simulink model "openManipulatorTorqueCtrlTask"  (R2021a)
settings: Solver=VariableStepAuto  StartTime=0.0  StopTime=3  RelTol=1e-3
PreLoadFcn:
  | openManipulatorParameters;
undefined symbols (not defined in the file): ctrlLowerLimit, ctrlUpperLimit, gripLowerLimit, gripUpperLimit, initPos, Kd, KdCart, Kfilt, KfiltCart, KiCart, KiGrip, KpCart, KpGrip, robot, TsCtrl, X, Y, Z
libraries: nesl_utility x26, sm_lib x23, OpenManipulatorLib x7, fl_lib x4, pid_lib x3, robotmaniplib x2, Multibody_Multiphysics_Lib x2
(part 2 of 2)

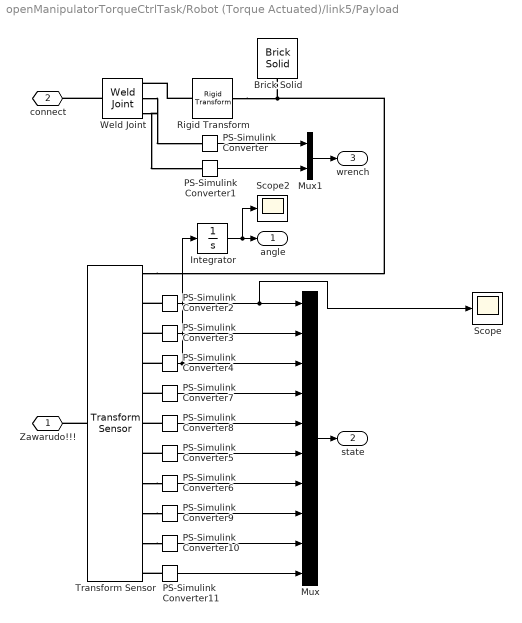
== system openManipulatorTorqueCtrlTask/Robot (Torque Actuated)/link5/Payload ==
  Brick Solid : sm_lib/Body Elements/Brick Solid  GraphicAmbientColor=[0.15 0.15 0.15 1.0]  BasedOnType=Density  BrickDimensions=[0.03 0.3 0.03]  BrickDimensionUnits=m  CenterOfMass=[0 0 0]  CenterOfMassUnits=m  GraphicDiffuseColor=[0.5 0.5 0.5]  Density=100  DensityUnits=kg/m^3  DoExposeReferenceFrame=on  GraphicEmissiveColor=[0.0 0.0 0.0 1.0]  ExportEntireGeometry=off  SerializedFrames=<Frames/>  MarkerShape=Sphere  MarkerSize=10  GraphicType=FromGeometry  InertiaType=CalculateFromGeometry  Mass=1  MassUnits=kg  MomentsOfInertia=[1 1 1]  MomentsOfInertiaUnits=kg*m^2  GraphicOpacity=1.0  ProductsOfInertia=[0 0 0]  ProductsOfInertiaUnits=kg*m^2  GraphicShininess=75  GraphicSpecularColor=[0.5 0.5 0.5 1.0]  GraphicVisPropType=SimpleVisualProperties
  Integrator : Integrator
  Mux : Mux  Inputs=10
  Mux1 : Mux  Inputs=2
  PS-Simulink Converter{,1..11} (12 alike) : nesl_utility/PS-Simulink Converter  PhysicalDomain=network_engine_domain  SubClassName=ps_output  LeftPortType=input  RightPortType=output  PseudoPeriodic=off  Frequencies=[]  Unit=inherit  AffineConversion=off
      settings: SourceProductBaseCode=PW,SS
  Rigid Transform : sm_lib/Frames and Transforms/Rigid Transform  TranslationMethod=StandardAxis  TranslationStandardOffset=0.2  TranslationLengthUnit=m  TranslationStandardAxis=+X  TranslationCartesianOffset=[0 0 0]  TranslationROffset=0  TranslationROffsetUnits=m  TranslationZOffset=0  TranslationZOffsetUnits=m  TranslationThetaOffset=0  TranslationThetaOffsetUnits=deg  RotationMethod=StandardAxis  RotationAngleUnits=deg  RotationStandardAxis=+Z  RotationAngle=90  RotationArbitraryAxis=[0 0 1]  FollAlignAxisA=+X  BaseAlignAxisA=+Y  FollAlignAxisB=+Y  BaseAlignAxisB=+Z  RotationSequenceAxes=FollowerAxes  RotationSequence=XYX  RotationSequenceAngles=[0 0 0]  RotationSequenceAnglesUnits=deg  RotationMatrix=[1 0 0; 0 1 0; 0 0 1]
  Scope : Scope
  Scope2 : Scope
  Transform Sensor : sm_lib/Frames and Transforms/Transform Sensor  MeasurementFrame=Base  SenseAngle=off  SenseAxis=off  SenseAngle1=off  SenseAngle2=off  SenseAngle3=off  SenseQ=on  SenseR=off  SenseOmegaX=on  SenseOmegaY=on  SenseOmegaZ=on  SenseOmega1=off  SenseOmega2=off  SenseOmega3=off  SenseQDot=off  SenseRDot=off  SenseAlphaX=off  SenseAlphaY=off  SenseAlphaZ=off  SenseAlpha1=off  SenseAlpha2=off  SenseAlpha3=off  SenseQDDot=off  SenseRDDot=off  SenseX=on  SenseY=on  SenseZ=on  SenseRad=off  SenseAzim=off  SenseDist=off  SenseInc=off  SenseXDot=on  SenseYDot=on  SenseZDot=on  SenseRadDot=off  SenseAzimDot=off  SenseDistDot=off  SenseIncDot=off  SenseXDDot=off  SenseYDDot=off  SenseZDDot=off  SenseRadDDot=off  SenseAzimDDot=off  SenseDistDDot=off  SenseIncDDot=off
  Weld Joint : sm_lib/Joints/Weld Joint  JointMode=Normal  SenseConstraintForce=off  SenseConstraintForceX=off  SenseConstraintForceY=off  SenseConstraintForceZ=off  SenseConstraintTorque=off  SenseConstraintTorqueX=off  SenseConstraintTorqueY=off  SenseConstraintTorqueZ=off  SenseTotalForce=on  SenseTotalForceX=off  SenseTotalForceY=off  SenseTotalForceZ=off  SenseTotalTorque=on  SenseTotalTorqueX=off  SenseTotalTorqueY=off  SenseTotalTorqueZ=off  CompositeWrenchDir=FollowerOnBase  CompositeWrenchFrame=BaseFrame
  Zawarudo!!! : PMIOPort  Side=Left
  connect : PMIOPort  Port=2  Side=Left
  angle : Outport
  state : Outport  Port=2
  wrench : Outport  Port=3
  wires:
  Integrator/1 -> Scope2/1, angle/1
  PS-Simulink Converter1/1 -> Mux1/2
  PS-Simulink Converter3/1 -> Mux/2
  PS-Simulink Converter5/1 -> Mux/6
  PS-Simulink Converter6/1 -> Mux/7
  PS-Simulink Converter4/1 -> Integrator/1, Mux/3
  PS-Simulink Converter8/1 -> Mux/5
  PS-Simulink Converter7/1 -> Mux/4
  Mux/1 -> state/1
  Mux1/1 -> wrench/1
  PS-Simulink Converter/1 -> Mux1/1
  PS-Simulink Converter11/1 -> Mux/10
  PS-Simulink Converter10/1 -> Mux/9
  PS-Simulink Converter9/1 -> Mux/8
  PS-Simulink Converter2/1 -> Scope/1, Mux/1
  connections:
  Rigid Transform/RConn1 -- Transform Sensor/RConn1 -- Brick Solid/RConn1
  Weld Joint/RConn2 -- PS-Simulink Converter/LConn1
  Rigid Transform/LConn1 -- Weld Joint/RConn1
  PS-Simulink Converter2/LConn1 -- Transform Sensor/RConn2
  Transform Sensor/LConn1 -- Zawarudo!!!/RConn1
  Weld Joint/LConn1 -- connect/RConn1
  PS-Simulink Converter3/LConn1 -- Transform Sensor/RConn3
  PS-Simulink Converter5/LConn1 -- Transform Sensor/RConn7
  Transform Sensor/RConn8 -- PS-Simulink Converter6/LConn1
  PS-Simulink Converter4/LConn1 -- Transform Sensor/RConn4
  PS-Simulink Converter8/LConn1 -- Transform Sensor/RConn6
  PS-Simulink Converter7/LConn1 -- Transform Sensor/RConn5
  PS-Simulink Converter11/LConn1 -- Transform Sensor/RConn11
  Transform Sensor/RConn10 -- PS-Simulink Converter10/LConn1
  Transform Sensor/RConn9 -- PS-Simulink Converter9/LConn1
  Weld Joint/RConn3 -- PS-Simulink Converter1/LConn1

== matlab function openManipulatorTorqueCtrlTask/Controller/MATLAB Function ==
  data: theta_o_hat input; theta_o input; xd input; Rd input; y output; a output; b output; c output; ref input; state input; dbg output
function [y,a, b, c, dbg] = fcn(theta_o_hat, theta_o, xd, Rd, ref, state)
%% gains
% ICL gain
N_o = 20
ICL_update = false
ICL_switcher = true
k_cl_m = 0.2
k_cl_rp = 0.2
k_cl_I = 0.2
k_cl_Izz = 0.3
k_cl_ri = 0.3
k_cl = [k_cl_m k_cl_rp*ones(1,3) k_cl_I*ones(1,5) k_cl_Izz k_cl_ri*ones(1,6)]
k_cl_gain = diag(k_cl)

% gamma o
g_m = 7.0
g_rp = 5.0
g_I = 0.23
g_Izz = 0.2
g_ri = 8.0
gg = [g_m g_rp*ones(1,3) g_I*ones(1,5) g_Izz g_ri*ones(1,6)]
g_o = diag(gg)

% Kd matrix
Kdl = 2
Kdr = 0.5
Kdd = [Kdl*ones(1,3) Kdr*ones(1,3)]
Kd = diag(Kdd)

% sliding parameter
lambda = 1.5

% deadband in which to stop adaptation
deadband = 0.003

%% function definition
function output = vee(matrix)
    output = [matrix(3, 2); matrix(1, 3); matrix(2, 1)];
end

function output = Pa(matrix)
    output = 0.5 * (matrix - matrix.');
end

function output = skew(v)
   output =  [    0 -v(3)   v(2)
               v(3)     0  -v(1)
              -v(2)  v(1)      0];
end

function output = L(v)
    output = [v(1)  v(2)  v(3)     0     0     0
                 0  v(1)     0  v(2)  v(3)     0
                 0     0  v(1)     0  v(2)  v(3)];
end
%% initialize


%% unpack ref
vd = [ref(1); ref(2); ref(3)];
wd = [ref(4); ref(5); ref(6)];

%% unpack state
quat = [state(1) state(2) state(3) state(4)];
R = quat2rotm(quat);
w = [state(5); state(6); state(7);]
x = [state(8); state(9); state(10);]
v = [state(11); state(12); state(13);]

%% compute error signals
Re = Rd.' * R;
we = w - wd;
sigma = we + lambda*Rd*vee(Pa(Re));
v_t = v - vd;
x_t = x - xd;
s = [v_t + lambda * x_t;
                  sigma];


y = state(1);
a = state(2);
b = state(3);
c = state(4);
dbg = 2;
end

== matlab function openManipulatorTorqueCtrlTask/Robot (Torque Actuated)/MATLAB Function ==
  data: w input; y output
function y = angle_gain(w)
y = -10*w;

== matlab function openManipulatorTorqueCtrlTask/Controller/Initialize Function/MATLAB Function ==
  data: theta_o_hat output; theta_o output; x_d output; Rd output size=[3,3]
function [theta_o_hat, theta_o, x_d, Rd] = fcn
% initial guess
theta_o_hat = zeros(10 + 3 * 2, 1);

% ground truth
mass = 0.027;
center_of_mass = [0 0 0];
inertia_matrix = [0.000204525 0 0 4.05e-06 0 0.000204525];
r = [-0.15 0.15];
theta_o = [mass mass*center_of_mass inertia_matrix r].';

Rd = [0 -1  0;
      1  0  0;
      0  0  1];

x_d = zeros(3, 1);
